simulink model "feedbackLin_Sensores_Noise"  (R2021a)
settings: Solver=ode1  StartTime=00  StopTime=100  FixedStep=0.005  RelTol=1e-3
values from neighbouring files (symbols this model uses):
  g = 9.31    [Metrics_Info.m]    (also in initEnv.m)
undefined symbols (not defined in the file or in its folder): Controller, DiscIntNeverNeededParam, Discrete, Earth, Estimator, gcbh, init, Rec, rho, SDTV, sensorCalibrationData, Sensors, States, Time, Ts, var_acc_angle_N, var_bias_gyr_N, var_gyro_p_N, Vehicle, vrmfunc, VTs, WGS84
libraries: simulink x26, ctrlSharedLib x4, sharedtransform x3, shared6dof x1, aerolibasang x1, dynamicsLibrary x1, aerolibtransform2 x1, aerolibnav x1, visionconversions x1, visiongeotforms x1
(part 2 of 3)

== system feedbackLin_Sensores_Noise/Subsystem2/Subsystem/State Estimator/SensorPreprocessing/sensordata_group ==
  HAL_acc_SI : Inport  OutDataTypeStr=Bus: HAL_acc_SI_t
  HAL_gyro_SI : Inport  Port=2  OutDataTypeStr=Bus: HAL_gyro_SI_t
  HAL_ultrasound_SI : Inport  Port=3  OutDataTypeStr=Bus: HAL_ultrasound_SI_t
  HAL_pressure_SI : Inport  Port=4  OutDataTypeStr=Bus: HAL_pressure_SI_t
  HAL_vbat_SI : Inport  Port=5  OutDataTypeStr=Bus: HAL_vbat_SI_t
  Bus Selector1 : BusSelector  OutputSignals=vbat_V,vbat_percentage
  Bus Selector3 : BusSelector  OutputSignals=x,y,z
  Bus Selector4 : BusSelector  OutputSignals=x,y,z,temperature
  Bus Selector5 : BusSelector  OutputSignals=altitude
  Bus Selector6 : BusSelector  OutputSignals=pressure
  Out Bus Element : Outport  VectorParamsAs1DForOutWhenUnconnected=off  PortName=sensordata_datin  Element=ddx
  Out Bus Element1 : Outport  VectorParamsAs1DForOutWhenUnconnected=off  PortName=sensordata_datin  Element=ddy
  Out Bus Element2 : Outport  VectorParamsAs1DForOutWhenUnconnected=off  PortName=sensordata_datin  Element=ddz
  Out Bus Element3 : Outport  VectorParamsAs1DForOutWhenUnconnected=off  PortName=sensordata_datin  Element=p
  Out Bus Element4 : Outport  VectorParamsAs1DForOutWhenUnconnected=off  PortName=sensordata_datin  Element=q
  Out Bus Element5 : Outport  VectorParamsAs1DForOutWhenUnconnected=off  PortName=sensordata_datin  Element=r
  Out Bus Element6 : Outport  VectorParamsAs1DForOutWhenUnconnected=off  PortName=sensordata_datin  Element=altitude_sonar
  Out Bus Element7 : Outport  VectorParamsAs1DForOutWhenUnconnected=off  PortName=sensordata_datin  Element=prs
  Out Bus Element8 : Outport  VectorParamsAs1DForOutWhenUnconnected=off  PortName=sensordata_datin  Element=vbat_V
  Out Bus Element9 : Outport  VectorParamsAs1DForOutWhenUnconnected=off  PortName=sensordata_datin  Element=vbat_percentage
  Out1 : Outport  Port=2
  wires:
  HAL_gyro_SI/1 -> Bus Selector4/1
  HAL_acc_SI/1 -> Bus Selector3/1
  HAL_pressure_SI/1 -> Bus Selector6/1
  HAL_ultrasound_SI/1 -> Bus Selector5/1
  Bus Selector4/1 -> Out Bus Element3/1  "<x>"
  Bus Selector3/3 -> Out Bus Element2/1  "<z>"
  Bus Selector4/3 -> Out Bus Element5/1  "<z>"
  Bus Selector5/1 -> Out Bus Element6/1  "<altitude>"
  Bus Selector6/1 -> Out Bus Element7/1  "<pressure>"
  Bus Selector4/2 -> Out Bus Element4/1  "<y>"
  Bus Selector3/1 -> Out Bus Element/1  "<x>"
  Bus Selector3/2 -> Out Bus Element1/1  "<y>"
  Bus Selector1/1 -> Out Bus Element8/1  "<vbat_V>"
  HAL_vbat_SI/1 -> Bus Selector1/1
  Bus Selector1/2 -> Out Bus Element9/1  "<vbat_percentage>"
  Bus Selector4/4 -> Out1/1  "<temperature>"

== system feedbackLin_Sensores_Noise/Subsystem2/Subsystem/State Estimator/XY Position Estimator/EstimatorVelocity ==
  opticalFlow_datin : Inport
  Z_estimin : Inport  Port=2  SampleTime=Ts
  sensorIMU_datin : Inport  Port=3
  orient_estimin : Inport  Port=4
  angular velocity : Inport  Port=5
  AccelerationHandling : Subsystem
  Angular velocity compensation for optical flow : Subsystem
  DataHandling : Subsystem
  Delay : Delay  DelayLength=1  InitialCondition=0
  KalmanFilter_dxdy : ctrlSharedLib/Kalman Filter  TimeDomain=Discrete-Time  UseCurrentEstimator=on  ModelSource=Individual A, B, C, D matrices  ModelSourceVariable=ss(0.95,1,1,0,1)  A=Estimator.pos.kfVelo.A  B=Estimator.pos.kfVelo.B  C=Estimator.pos.kfVelo.C  D=Estimator.pos.kfVelo.D  NumberOfStates=1  NumberOfInputs=1  NumberOfOutputs=1  InitialEstimateSource=Dialog  X0=0  P0=10  UseK=off  UseGH=off  NumberOfProcessNoiseInputs=1  G=Estimator.pos.kfVelo.G  TimeInvariantG=on  H=Estimator.pos.kfVelo.H  TimeInvariantH=on  Q=Estimator.pos.kfVelo.Q  TimeInvariantQ=on  R=Estimator.pos.kfVelo.R  TimeInvariantR=on  N=Estimator.pos.kfVelo.N  TimeInvariantN=on  AddInputPort=on  AddEnablePort=on  OutputEstimatedY=off  OutputP=off  Ts=-1
  Selector1 : Selector  InputPortWidth=4  IndexOptions=Index vector (dialog)  Indices=[1 2]  OutputSizes=1
  XY velocity w/o angular velocity compensation : Subsystem
  Z_estimin1 : InportShadow  Port=2  SampleTime=Ts
  angular velocity compensation : Sum
  dxy_estimout : Outport  VectorParamsAs1DForOutWhenUnconnected=off
  wires:
  Z_estimin/1 -> DataHandling/1(Z_estimin), AccelerationHandling/4(Z_estimin)
  KalmanFilter_dxdy/1 -> Selector1/1
  sensorIMU_datin/1 -> AccelerationHandling/2(sensorIMU_datin), DataHandling/3(sensorIMU_datin)
  orient_estimin/1 -> AccelerationHandling/3(orient_estimin), DataHandling/2(orient_estimin)
  Z_estimin1/1 -> XY velocity w/o angular velocity compensation/2(z_estimate), Angular velocity compensation for optical flow/1(z_estimate)
  AccelerationHandling/1(acceleration_world) -> KalmanFilter_dxdy/1
  angular velocity compensation/1 -> KalmanFilter_dxdy/2
  Delay/1 -> DataHandling/5(dxyOF_datin)
  Selector1/1 -> dxy_estimout/1, Delay/1
  angular velocity/1 -> Angular velocity compensation for optical flow/2(Angular velocity w/o bias)
  Angular velocity compensation for optical flow/1(angular velocity correction) -> angular velocity compensation/2
  XY velocity w/o angular velocity compensation/1(optical_flow_dx_dy) -> DataHandling/4(dxy_estimin), AccelerationHandling/1(dxy_estimin), angular velocity compensation/1
  opticalFlow_datin/1 -> XY velocity w/o angular velocity compensation/1(optical_flow)
  DataHandling/1(enable_flag) -> KalmanFilter_dxdy/3

== system feedbackLin_Sensores_Noise/Subsystem2/Subsystem/State Estimator/XY Position Estimator/EstimatorXYPosition ==
  note: Switching from orientationControl to Position
      | control reset the current world position estimate
      | (happens when using no markers)
  dxy_estimin : Inport
  orient_estimin : Inport  Port=2  SampleTime=Ts
  controlModePosVSOrient_flagin : Inport  Port=3
  dz_estimin : Inport  Port=4
  Math Function : Math  Operator=transpose  SignedPower=on  SaturateOnIntegerOverflow=on
  Mux2 : Mux  Inputs=2
  Product : Product  Multiplication=Matrix(*)
  Rotation Angles to Direction Cosine Matrix : sharedtransform/Rotation Angles to Direction Cosine Matrix  rotationOrder=ZYX  aMode=aMode
      settings: SourceProductBaseCode=AE,PW,DR,MT,UV,VE
  Scope : Scope
  SelectdXY : Selector  InputPortWidth=3  IndexOptions=Index vector (dialog)  Indices=[1 2]  OutputSizes=1
  SimplyIntegrateVelocity : DiscreteIntegrator  ExternalReset=rising  SampleTime=Ts  ICPrevOutput=DiscIntNeverNeededParam  ICPrevScaledInput=DiscIntNeverNeededParam
  XY_estimout : Outport  VectorParamsAs1DForOutWhenUnconnected=off
  wires:
  controlModePosVSOrient_flagin/1 -> SimplyIntegrateVelocity/2
  Product/1 -> SelectdXY/1
  Mux2/1 -> Product/2
  dz_estimin/1 -> Mux2/2
  SimplyIntegrateVelocity/1 -> XY_estimout/1
  dxy_estimin/1 -> Mux2/1
  orient_estimin/1 -> Rotation Angles to Direction Cosine Matrix/1
  Rotation Angles to Direction Cosine Matrix/1 -> Math Function/1
  SelectdXY/1 -> Scope/1, SimplyIntegrateVelocity/1
  Math Function/1 -> Product/1

== system feedbackLin_Sensores_Noise/Subsystem2/Subsystem/Sensors Model/Sensors (Dynamics)/Sensor System/Camera ==
  note: Optical flow is measured by using a camera and is calculated based on how the image actually moves. It is thus dependant on body angular velocity and body's linear velocity.
  note: This is a crude simulation of "optical flow" (vx,vy,vz) as
      | fed into the c-function rsedu_optical_flow() on the Rolling Spider
      | by internal, inaccessible code of Parrot's firmware.
      | This is assumed to be far from what "optical flow (vx,vy,vz)" actually is!
  states : Inport  OutDataTypeStr=Bus: StatesBus
  Add1 : Sum
  Bus Selector1 : BusSelector  OutputSignals=V_body
  Bus Selector3 : BusSelector  OutputSignals=X_ned
  Bus Selector4 : BusSelector  OutputSignals=Omega_body
  Data Type Conversion : DataTypeConversion  OutDataTypeStr=single
  Demux4 : Demux  Outputs=2
  Divide : Product  Inputs=*/
  Gain1 : Gain  Gain=0.8*[-1,1]
  Gain2 : Gain  Gain=-1
  Mux7 : Mux  Inputs=2
  Mux8 : Mux  Inputs=2
  Product : Product
  Product1 : Product
  Reshape : Reshape
  Select dx,dy : Selector  InputPortWidth=3  IndexOptions=Index vector (dialog)  Indices=[1 2]  OutputSizes=1
  Select dx,dy1 : Selector  InputPortWidth=3  IndexOptions=Index vector (dialog)  Indices=[1 2]  OutputSizes=1
  Select dz : Selector  InputPortWidth=3  IndexOptions=Index vector (dialog)  Indices=3  OutputSizes=1
  Select dz1 : Selector  InputPortWidth=3  IndexOptions=Index vector (dialog)  Indices=3  OutputSizes=1
  SwitchPlanarOpticalFlow : Selector  InputPortWidth=2  IndexOptions=Index vector (dialog)  Indices=[2 1]  OutputSizes=1
  VelocityToOpticalFlow_Gain : Gain  Gain=Sensors.velocityToOpticalFlowGain
  opticalFlow_datout : Outport  VectorParamsAs1DForOutWhenUnconnected=off
  wires:
  SwitchPlanarOpticalFlow/1 -> Add1/2
  Select dz/1 -> Mux8/2
  Bus Selector3/1 -> Select dz1/1  "<X_ned>"
  Mux7/1 -> SwitchPlanarOpticalFlow/1
  Bus Selector4/1 -> Reshape/1  "<Omega_body>"
  VelocityToOpticalFlow_Gain/1 -> Data Type Conversion/1
  Select dx,dy/1 -> Add1/1
  Reshape/1 -> Select dx,dy1/1
  Data Type Conversion/1 -> opticalFlow_datout/1
  Gain2/1 -> Divide/2, Product1/2, Product/2
  Divide/1 -> Mux8/1
  Product1/1 -> Mux7/2
  Select dx,dy1/1 -> Gain1/1
  Product/1 -> Mux7/1
  Demux4/1 -> Product/1
  Gain1/1 -> Demux4/1
  Select dz1/1 -> Gain2/1
  Bus Selector1/1 -> Select dz/1, Select dx,dy/1  "<V_body>"
  Demux4/2 -> Product1/1
  Mux8/1 -> VelocityToOpticalFlow_Gain/1
  states/1 -> Bus Selector1/1, Bus Selector4/1, Bus Selector3/1
  Add1/1 -> Divide/1

== system feedbackLin_Sensores_Noise/Subsystem2/Subsystem/Sensors Model/Sensors (Dynamics)/Sensor System/IMU_Pressure ==
  note: IMU block simulates the 6DOF sensor MPU6050 that we have on board. Please note that this model cannot simulate the gyro's bias change over time!
  States : Inport
  Environment : Inport  Port=2
  Assumes takeoff was level1 : Bias  Bias=Sensors.altToPrsBias
  Bus Selector : BusSelector  OutputSignals=Accel_body,Omega_body,dOmega_body,DCM_be,X_ned
  Bus Selector1 : BusSelector  OutputSignals=Gravity_ned
  CG location : Constant  Value=Sensors.IMU.cg
  Data Type Conversion{,1..4} (5 alike) : DataTypeConversion  OutDataTypeStr=single
  Demux : Demux  Outputs=3
  Demux2 : Demux  Outputs=3
  HAL_acquisition_creator : Subsystem
  Mux : Mux  Inputs=8
  Product : Product  Multiplication=Matrix(*)
  Saturation : Saturate  UpperLimit=inf  LowerLimit=Sensors.altSensorMin  OutDataTypeStr=single
  Selector2 : Selector  InputPortWidth=3  IndexOptions=Index vector (dialog)  Indices=[3]  OutputSizes=1
  Three-axis Inertial Measurement Unit : aerolibnav/Three-axis Inertial Measurement Unit  units=Metric (MKS)  imu=Sensors.IMU.location  i_Ts=Ts  dtype_a=off  w_a=.7  z_a=.2  a_sf_cc=Sensors.IMU.accScaleCross  a_bias=Sensors.IMU.accBias  a_sat=Sensors.IMU.accLimits  dtype_g=off  w_g=.7  z_g=.2  g_sf_cc=Sensors.IMU.gyroScaleCross  g_bias=Sensors.IMU.gyroBias  g_sens=Sensors.IMU.gyroGBias  g_sat=Sensors.IMU.gyroLimits  i_rand=on  i_seeds=Sensors.IMU.noiseSeeds  i_pow=Sensors.IMU.noisePower
  altToprs_gain : Gain  Gain=Sensors.altToPrsGain  ParamDataTypeStr=single  OutDataTypeStr=single
  altToprs_gain1 : Gain  Gain=-1  ParamDataTypeStr=single  OutDataTypeStr=single
  sensordata_datout : Outport  OutDataTypeStr=Bus: HAL_acquisition_t  VectorParamsAs1DForOutWhenUnconnected=off
  wires:
  altToprs_gain1/1 -> Saturation/1
  Data Type Conversion4/1 -> Mux/8
  Data Type Conversion3/1 -> Mux/7
  Data Type Conversion2/1 -> Demux2/1
  Data Type Conversion/1 -> Demux/1
  Assumes takeoff was level1/1 -> Data Type Conversion4/1
  Bus Selector/5 -> Selector2/1  "<X_ned>"
  States/1 -> Bus Selector/1
  Product/1 -> Three-axis Inertial Measurement Unit/5
  Bus Selector1/1 -> Product/2  "<Gravity_ned>"
  Bus Selector/4 -> Product/1  "<DCM_be>"
  CG location/1 -> Three-axis Inertial Measurement Unit/4
  Bus Selector/3 -> Three-axis Inertial Measurement Unit/3  "<dOmega_body>"
  Environment/1 -> Bus Selector1/1
  Bus Selector/2 -> Three-axis Inertial Measurement Unit/2  "<Omega_body>"
  Bus Selector/1 -> Three-axis Inertial Measurement Unit/1  "<Accel_body>"
  HAL_acquisition_creator/1(HAL_acquisition_t) -> sensordata_datout/1
  Data Type Conversion1/1 -> HAL_acquisition_creator/1(sensors)
  Three-axis Inertial Measurement Unit/2 -> Data Type Conversion2/1
  Three-axis Inertial Measurement Unit/1 -> Data Type Conversion/1
  Mux/1 -> Data Type Conversion1/1
  altToprs_gain/1 -> Assumes takeoff was level1/1  "prs"
  Saturation/1 -> Data Type Conversion3/1  "altitude_sonar"
  Selector2/1 -> altToprs_gain/1, altToprs_gain1/1
  Demux/3 -> Mux/3  "ddz"
  Demux2/3 -> Mux/6  "r"
  Demux/2 -> Mux/2  "ddy"
  Demux/1 -> Mux/1  "ddx"
  Demux2/1 -> Mux/4  "p"
  Demux2/2 -> Mux/5  "q"

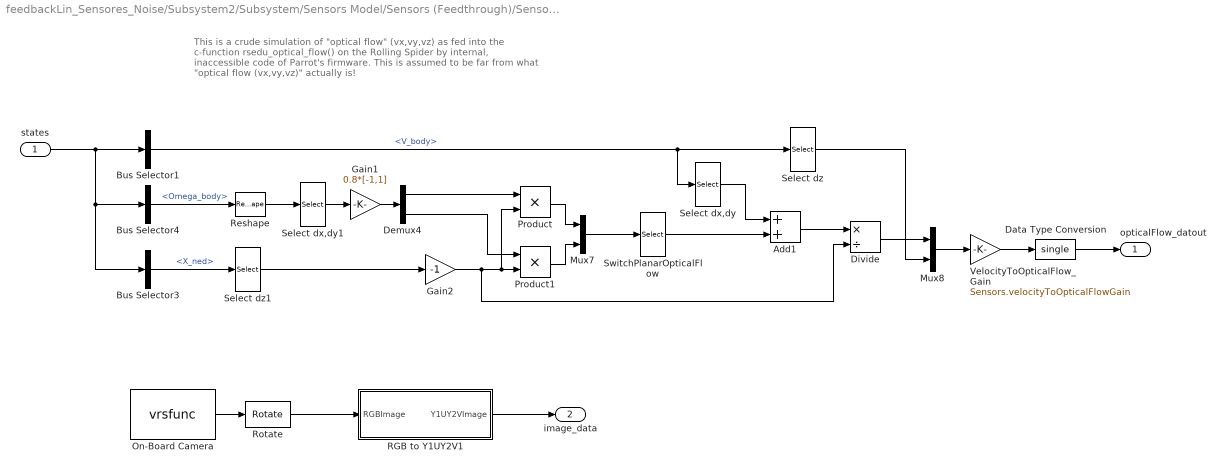
== system feedbackLin_Sensores_Noise/Subsystem2/Subsystem/Sensors Model/Sensors (Feedthrough)/Sensor System/Camera ==
  note: This is a crude simulation of "optical flow" (vx,vy,vz) as
      | fed into the c-function rsedu_optical_flow() on the Rolling Spider
      | by internal, inaccessible code of Parrot's firmware.
      | This is assumed to be far from what "optical flow (vx,vy,vz)" actually is!
  states : Inport  OutDataTypeStr=Bus: StatesBus
  Add1 : Sum
  Bus Selector1 : BusSelector  OutputSignals=V_body
  Bus Selector3 : BusSelector  OutputSignals=X_ned
  Bus Selector4 : BusSelector  OutputSignals=Omega_body
  Data Type Conversion : DataTypeConversion  OutDataTypeStr=single
  Demux4 : Demux  Outputs=2
  Divide : Product  Inputs=*/
  Gain1 : Gain  Gain=0.8*[-1,1]
  Gain2 : Gain  Gain=-1
  Mux7 : Mux  Inputs=2
  Mux8 : Mux  Inputs=2
  On-Board Camera : S-Function  InstantiateOnLoad=on  LoadFcn=vrmfunc('FnLoad', gcbh);  InitFcn=""  StartFcn=vrmfunc('FnSimStatus', gcbh, 'running')  StopFcn=vrmfunc('FnStop', gcbh)  FunctionName=vrsfunc  Parameters=SampleTime, VideoDimensions, false  SFunctionDeploymentMode=off  EnableBusSupport=off  mask(Virtual Reality Sink){SampleTime=VTs, ViewEnable=on, RemoteChange=off, RemoteView=off, FieldsWritten=, WorldFileName=asbQuadcopterWorld.wrl, WorldDescription=, AutoView=off, VideoDimensions=[160 120], AllowVariableSize=off, FigureProperties=}
      mask prompts: SampleTime "Sample Time"; ViewEnable "View"; RemoteChange "Remote Change"; RemoteView "Remote View"; FieldsWritten "Fields Written"; WorldFileName "World File Name"; WorldDescription "World Description"; VideoDimensions "Video Dimensions"; AllowVariableSize "Allow Variable Size"; FigureProperties "Figure Properties"
      mask help: Controls the selected fields of a virtual world according to given inputs.
      mask init:
      | set_param(gcbh, 'MaskDisplay', vrmfunc('FnIcon'));
      settings: CopyFcn=vrmfunc('FnCopy', gcbh);  DeleteFcn=vrmfunc('FnDelete', gcbh);  PreSaveFcn=vrmfunc('FnPreSave', gcbh);  PauseFcn=vrmfunc('FnSimStatus', gcbh, 'paused');  ContinueFcn=vrmfunc('FnSimStatus', gcbh, 'running');  DestroyFcn=vrmfunc('FnDestroy', gcbh);  OpenFcn=vrmfunc('FnOpen', gcbh);  CloseFcn=vrmfunc('FnClose', gcbh);
      mask Help: helpview(vrmfunc('FnHelpTopic'), 'vr_vrtovideo');
      mask Display: image(imread('vrblockicon.png'));
  Product : Product
  Product1 : Product
  RGB to Y1UY2V1 : Subsystem
  Reshape : Reshape
  Rotate : visiongeotforms/Rotate  outSizeR=Expanded to fit rotated input image  src_angle=Specify via dialog  unit_angle=Degrees  angle=pi/2  maxAngle=pi  dispImage=Top-left corner  method=Table lookup  fillVal=0  interpMethod=Bilinear  roundingMode=Nearest  overflowMode=on  prodOutputMode=Binary point scaling  prodOutputWordLength=32  prodOutputFracLength=10
  Select dx,dy : Selector  InputPortWidth=3  IndexOptions=Index vector (dialog)  Indices=[1 2]  OutputSizes=1
  Select dx,dy1 : Selector  InputPortWidth=3  IndexOptions=Index vector (dialog)  Indices=[1 2]  OutputSizes=1
  Select dz : Selector  InputPortWidth=3  IndexOptions=Index vector (dialog)  Indices=3  OutputSizes=1
  Select dz1 : Selector  InputPortWidth=3  IndexOptions=Index vector (dialog)  Indices=3  OutputSizes=1
  SwitchPlanarOpticalFlow : Selector  InputPortWidth=2  IndexOptions=Index vector (dialog)  Indices=[2 1]  OutputSizes=1
  VelocityToOpticalFlow_Gain : Gain  Gain=Sensors.velocityToOpticalFlowGain
  opticalFlow_datout : Outport  VectorParamsAs1DForOutWhenUnconnected=off
  image_data : Outport  Port=2  VectorParamsAs1DForOutWhenUnconnected=off
  wires:
  states/1 -> Bus Selector1/1, Bus Selector4/1, Bus Selector3/1
  Demux4/2 -> Product1/1
  Demux4/1 -> Product/1
  Bus Selector1/1 -> Select dz/1, Select dx,dy/1  "<V_body>"
  Rotate/1 -> RGB to Y1UY2V1/1(RGBImage)
  Gain1/1 -> Demux4/1
  Add1/1 -> Divide/1
  Product/1 -> Mux7/1
  Select dz1/1 -> Gain2/1
  On-Board Camera/1 -> Rotate/1
  Select dx,dy1/1 -> Gain1/1
  Gain2/1 -> Divide/2, Product1/2, Product/2
  Reshape/1 -> Select dx,dy1/1
  Divide/1 -> Mux8/1
  Data Type Conversion/1 -> opticalFlow_datout/1
  RGB to Y1UY2V1/1(Y1UY2VImage) -> image_data/1
  VelocityToOpticalFlow_Gain/1 -> Data Type Conversion/1
  Product1/1 -> Mux7/2
  Mux7/1 -> SwitchPlanarOpticalFlow/1
  Mux8/1 -> VelocityToOpticalFlow_Gain/1
  Select dx,dy/1 -> Add1/1
  Bus Selector4/1 -> Reshape/1  "<Omega_body>"
  Select dz/1 -> Mux8/2
  Bus Selector3/1 -> Select dz1/1  "<X_ned>"
  SwitchPlanarOpticalFlow/1 -> Add1/2

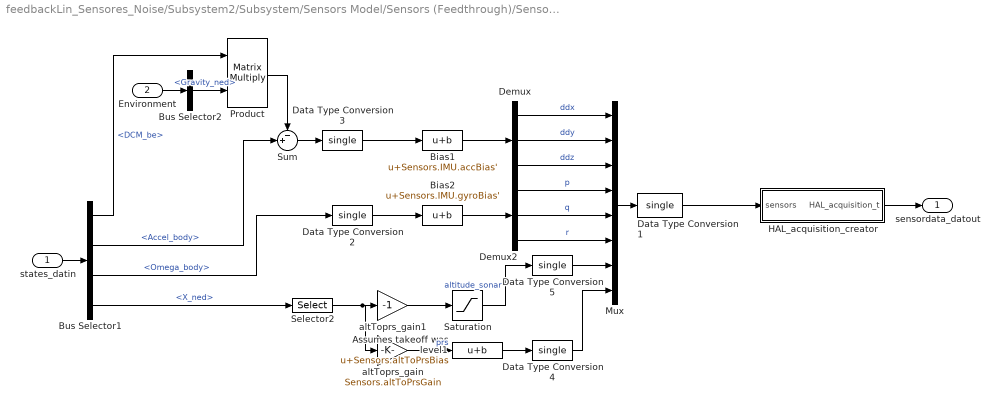
== system feedbackLin_Sensores_Noise/Subsystem2/Subsystem/Sensors Model/Sensors (Feedthrough)/Sensor System/IMU_Pressure ==
  states_datin : Inport  OutDataTypeStr=Bus: StatesBus
  Environment : Inport  Port=2
  Assumes takeoff was level1 : Bias  Bias=Sensors.altToPrsBias
  Bias1 : Bias  Bias=Sensors.IMU.accBias'
  Bias2 : Bias  Bias=Sensors.IMU.gyroBias'
  Bus Selector1 : BusSelector  OutputSignals=DCM_be,Accel_body,Omega_body,X_ned
  Bus Selector2 : BusSelector  OutputSignals=Gravity_ned
  Data Type Conversion{1..5} (5 alike) : DataTypeConversion  OutDataTypeStr=single
  Demux : Demux  Outputs=3
  Demux2 : Demux  Outputs=3
  HAL_acquisition_creator : Subsystem
  Mux : Mux  Inputs=8
  Product : Product  Multiplication=Matrix(*)
  Saturation : Saturate  UpperLimit=inf  LowerLimit=Sensors.altSensorMin  OutDataTypeStr=single
  Selector2 : Selector  InputPortWidth=3  IndexOptions=Index vector (dialog)  Indices=[3]  OutputSizes=1
  Sum : Sum  Inputs=-+|
  altToprs_gain : Gain  Gain=Sensors.altToPrsGain  ParamDataTypeStr=single  OutDataTypeStr=single
  altToprs_gain1 : Gain  Gain=-1  ParamDataTypeStr=single  OutDataTypeStr=single
  sensordata_datout : Outport  OutDataTypeStr=Bus: HAL_acquisition_t  VectorParamsAs1DForOutWhenUnconnected=off
  wires:
  Bias2/1 -> Demux2/1
  Bias1/1 -> Demux/1
  Product/1 -> Sum/1
  Bus Selector1/2 -> Sum/2  "<Accel_body>"
  Sum/1 -> Data Type Conversion3/1
  Bus Selector1/1 -> Product/1  "<DCM_be>"
  Bus Selector2/1 -> Product/2  "<Gravity_ned>"
  altToprs_gain1/1 -> Saturation/1
  Data Type Conversion5/1 -> Mux/7
  Data Type Conversion4/1 -> Mux/8
  Data Type Conversion2/1 -> Bias2/1
  Data Type Conversion3/1 -> Bias1/1
  Assumes takeoff was level1/1 -> Data Type Conversion4/1
  Bus Selector1/4 -> Selector2/1  "<X_ned>"
  states_datin/1 -> Bus Selector1/1
  Environment/1 -> Bus Selector2/1
  Bus Selector1/3 -> Data Type Conversion2/1  "<Omega_body>"
  HAL_acquisition_creator/1(HAL_acquisition_t) -> sensordata_datout/1
  Data Type Conversion1/1 -> HAL_acquisition_creator/1(sensors)
  Mux/1 -> Data Type Conversion1/1
  altToprs_gain/1 -> Assumes takeoff was level1/1  "prs"
  Saturation/1 -> Data Type Conversion5/1  "altitude_sonar"
  Selector2/1 -> altToprs_gain1/1, altToprs_gain/1
  Demux/3 -> Mux/3  "ddz"
  Demux2/3 -> Mux/6  "r"
  Demux/2 -> Mux/2  "ddy"
  Demux/1 -> Mux/1  "ddx"
  Demux2/1 -> Mux/4  "p"
  Demux2/2 -> Mux/5  "q"

== system feedbackLin_Sensores_Noise/Subsystem2/Subsystem/State Estimator/SensorPreprocessing/Temperature Compensation/Triggered Subsystem ==
  In1 : Inport
  Trigger : TriggerPort  TriggerType=either  VariantControl=Variant
  Out1 : Outport
  wires:
  In1/1 -> Out1/1

== system feedbackLin_Sensores_Noise/Subsystem2/Subsystem/State Estimator/XY Position Estimator/EstimatorVelocity/AccelerationHandling ==
  dxy_estimin : Inport
  sensorIMU_datin : Inport  Port=2
  orient_estimin : Inport  Port=3
  Z_estimin : Inport  Port=4
  Add : Sum  Inputs=-+
  Bus Selector1 : BusSelector  OutputSignals=ddx,ddy,ddz
  Deactivate Acceleration If OF is not used due to low altitude : simulink/Logic and Bit Operations/Compare To Constant  relop=<=  const=Estimator.pos.opticalFlowZMax  OutDataTypeStr=boolean
  Logical Operator : Logic  Operator=OR  AllPortsSameDT=off  OutDataTypeStr=boolean
  Mux6 : Mux  Inputs=3
  Product : Product  Inputs=3
  Product1 : Product  Multiplication=Matrix(*)
  Rotation Angles to Direction Cosine Matrix : sharedtransform/Rotation Angles to Direction Cosine Matrix  rotationOrder=ZYX  aMode=aMode
      settings: SourceProductBaseCode=AE,PW,DR,MT,UV,VE
  SelectPlanarddxy : Selector  InputPortWidth=3  IndexOptions=Index vector (dialog)  Indices=[1 2]  OutputSizes=1
  Selector : Selector  InputPortWidth=2  IndexOptions=Index vector (dialog)  Indices=1  OutputSizes=1
  Selector1 : Selector  InputPortWidth=2  IndexOptions=Index vector (dialog)  Indices=2  OutputSizes=1
  do not use acc if optical flow never available (Note OF@60Hz but ZOH to 200!) : simulink/Logic and Bit Operations/Compare To Constant  relop=~=  const=0  OutDataTypeStr=boolean
  do not use acc if optical flow never available (Note OF@60Hz but ZOH to 200!)1 : simulink/Logic and Bit Operations/Compare To Constant  relop=~=  const=0  OutDataTypeStr=boolean
  gainaccinput1 : Gain  OutDataTypeStr=single
  gravity : Constant  Value=[0 0 -g]
  acceleration_world : Outport  OutDataTypeStr=single  VectorParamsAs1DForOutWhenUnconnected=off
  wires:
  do not use acc if optical flow never available (Note OF@60Hz but ZOH to 200!)1/1 -> Logical Operator/2
  do not use acc if optical flow never available (Note OF@60Hz but ZOH to 200!)/1 -> Logical Operator/1
  Logical Operator/1 -> Product/1
  Selector1/1 -> do not use acc if optical flow never available (Note OF@60Hz but ZOH to 200!)1/1
  Selector/1 -> do not use acc if optical flow never available (Note OF@60Hz but ZOH to 200!)/1
  dxy_estimin/1 -> Selector1/1, Selector/1
  Product/1 -> acceleration_world/1
  Deactivate Acceleration If OF is not used due to low altitude/1 -> Product/3
  Z_estimin/1 -> Deactivate Acceleration If OF is not used due to low altitude/1
  Add/1 -> SelectPlanarddxy/1
  Product1/1 -> Add/1
  gravity/1 -> Product1/2
  SelectPlanarddxy/1 -> gainaccinput1/1
  Bus Selector1/3 -> Mux6/3  "<ddz>"
  Bus Selector1/1 -> Mux6/1  "<ddx>"
  sensorIMU_datin/1 -> Bus Selector1/1
  Mux6/1 -> Add/2
  Bus Selector1/2 -> Mux6/2  "<ddy>"
  orient_estimin/1 -> Rotation Angles to Direction Cosine Matrix/1
  Rotation Angles to Direction Cosine Matrix/1 -> Product1/1
  gainaccinput1/1 -> Product/2

== system feedbackLin_Sensores_Noise/Subsystem2/Subsystem/State Estimator/XY Position Estimator/EstimatorVelocity/Angular velocity compensation for optical flow ==
  note: Optical flow readings are affected by both linear and angular velocity of the drone. We need to subtract the effect of angular velocity before using the flow data
  z_estimate : Inport
  Angular velocity w/o bias : Inport  Port=2
  Abs : Abs
  Data Type Conversion : DataTypeConversion
  Demux : Demux  Outputs=2
  Gain1 : Gain  Gain=-1
  Mux : Mux  Inputs=2
  Selector : Selector  InputPortWidth=3  IndexOptions=Index vector (dialog)  Indices=[1 2]  OutputSizes=1
  prod : Product  Inputs=**
  angular velocity correction : Outport
  wires:
  Gain1/1 -> Mux/1
  Mux/1 -> Data Type Conversion/1
  Demux/2 -> Gain1/1
  Data Type Conversion/1 -> angular velocity correction/1
  prod/1 -> Demux/1
  z_estimate/1 -> Abs/1
  Demux/1 -> Mux/2
  Selector/1 -> prod/2
  Abs/1 -> prod/1
  Angular velocity w/o bias/1 -> Selector/1

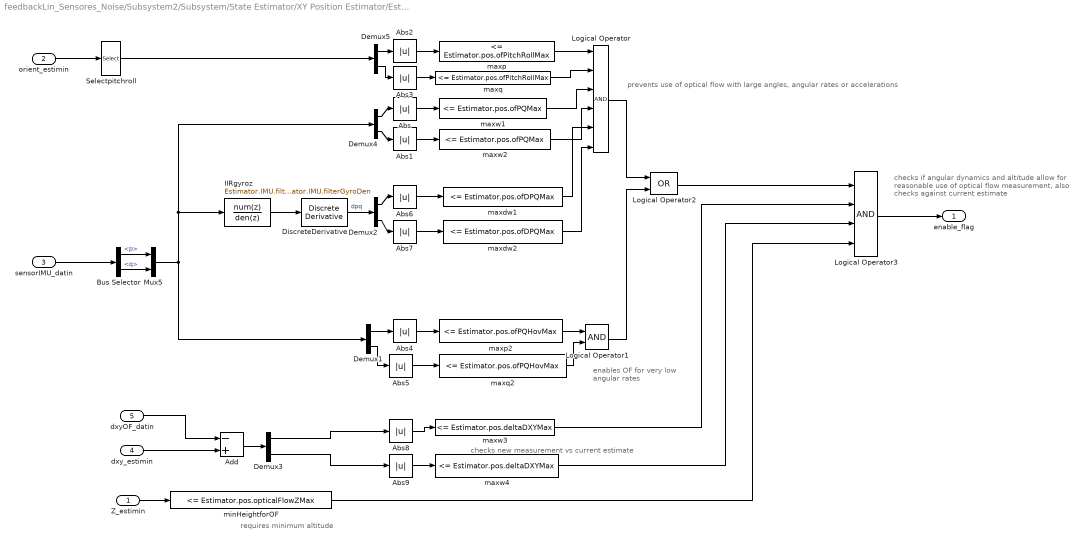
== system feedbackLin_Sensores_Noise/Subsystem2/Subsystem/State Estimator/XY Position Estimator/EstimatorVelocity/DataHandling ==
  note: prevents use of optical flow with large angles, angular rates or accelerations
  note: enables OF for very
      | low angular rates
  note: checks if angular dynamics and altitude allow for
      | reasonable use of optical flow measurement,
      | also checks against current estimate
  note: checks new measurement vs current estimate
  note: requires minimum altitude
  Z_estimin : Inport
  orient_estimin : Inport  Port=2
  sensorIMU_datin : Inport  Port=3
  dxy_estimin : Inport  Port=4
  dxyOF_datin : Inport  Port=5
  Abs{,1..9} (10 alike) : Abs
  Add : Sum  Inputs=-+
  Bus Selector : BusSelector  OutputSignals=p,q
  Demux{1..5} (5 alike) : Demux  Outputs=2
  DiscreteDerivative : simulink/Discrete/Discrete Derivative  gainval=1.0  ICPrevScaledInput=0.0  OutMin=[]  OutMax=[]  OutDataType=fixdt(1, 16)  OutScaling=2^-10  DoSatur=off
  IIRgyroz : DiscreteFilter  Numerator=Estimator.IMU.filterGyroNum  Denominator=Estimator.IMU.filterGyroDen
  Logical Operator : Logic  Inputs=6  AllPortsSameDT=off  OutDataTypeStr=boolean
  Logical Operator1 : Logic  AllPortsSameDT=off  OutDataTypeStr=boolean
  Logical Operator2 : Logic  Operator=OR  AllPortsSameDT=off  OutDataTypeStr=boolean
  Logical Operator3 : Logic  Inputs=4  AllPortsSameDT=off  OutDataTypeStr=boolean
  Mux5 : Mux  Inputs=2
  Selectpitchroll : Selector  InputPortWidth=3  IndexOptions=Index vector (dialog)  Indices=[2 3]  OutputSizes=1
  maxdw1 : simulink/Logic and Bit Operations/Compare To Constant  relop=<=  const=Estimator.pos.ofDPQMax  OutDataTypeStr=boolean
  maxdw2 : simulink/Logic and Bit Operations/Compare To Constant  relop=<=  const=Estimator.pos.ofDPQMax  OutDataTypeStr=boolean
  maxp : simulink/Logic and Bit Operations/Compare To Constant  relop=<=  const=Estimator.pos.ofPitchRollMax  OutDataTypeStr=boolean
  maxp2 : simulink/Logic and Bit Operations/Compare To Constant  relop=<=  const=Estimator.pos.ofPQHovMax  OutDataTypeStr=boolean
  maxq : simulink/Logic and Bit Operations/Compare To Constant  relop=<=  const=Estimator.pos.ofPitchRollMax  OutDataTypeStr=boolean
  maxq2 : simulink/Logic and Bit Operations/Compare To Constant  relop=<=  const=Estimator.pos.ofPQHovMax  OutDataTypeStr=boolean
  maxw1 : simulink/Logic and Bit Operations/Compare To Constant  relop=<=  const=Estimator.pos.ofPQMax  OutDataTypeStr=boolean
  maxw2 : simulink/Logic and Bit Operations/Compare To Constant  relop=<=  const=Estimator.pos.ofPQMax  OutDataTypeStr=boolean
  maxw3 : simulink/Logic and Bit Operations/Compare To Constant  relop=<=  const=Estimator.pos.deltaDXYMax  OutDataTypeStr=boolean
  maxw4 : simulink/Logic and Bit Operations/Compare To Constant  relop=<=  const=Estimator.pos.deltaDXYMax  OutDataTypeStr=boolean
  minHeightforOF : simulink/Logic and Bit Operations/Compare To Constant  relop=<=  const=Estimator.pos.opticalFlowZMax  OutDataTypeStr=boolean
  enable_flag : Outport  VectorParamsAs1DForOutWhenUnconnected=off
  wires:
  minHeightforOF/1 -> Logical Operator3/4
  IIRgyroz/1 -> DiscreteDerivative/1
  Mux5/1 -> Demux1/1, Demux4/1, IIRgyroz/1
  maxw4/1 -> Logical Operator3/3
  maxw3/1 -> Logical Operator3/2
  dxyOF_datin/1 -> Add/1
  Demux3/2 -> Abs9/1
  Demux3/1 -> Abs8/1
  dxy_estimin/1 -> Add/2
  Add/1 -> Demux3/1
  Abs9/1 -> maxw4/1
  Abs8/1 -> maxw3/1
  Logical Operator2/1 -> Logical Operator3/1
  Logical Operator3/1 -> enable_flag/1
  DiscreteDerivative/1 -> Demux2/1  "dpq"
  Demux2/2 -> Abs7/1
  Demux2/1 -> Abs6/1
  Abs7/1 -> maxdw2/1
  Abs6/1 -> maxdw1/1
  Logical Operator1/1 -> Logical Operator2/2
  Demux1/2 -> Abs5/1
  Demux1/1 -> Abs4/1
  Abs5/1 -> maxq2/1
  Abs4/1 -> maxp2/1
  Abs3/1 -> maxq/1
  Abs2/1 -> maxp/1
  Demux4/2 -> Abs1/1
  Demux4/1 -> Abs/1
  Abs1/1 -> maxw2/1
  Abs/1 -> maxw1/1
  Z_estimin/1 -> minHeightforOF/1
  Logical Operator/1 -> Logical Operator2/1
  maxw1/1 -> Logical Operator/3
  Bus Selector/1 -> Mux5/1  "<p>"
  Selectpitchroll/1 -> Demux5/1
  sensorIMU_datin/1 -> Bus Selector/1
  maxq2/1 -> Logical Operator1/2
  Bus Selector/2 -> Mux5/2  "<q>"
  maxp/1 -> Logical Operator/1
  maxw2/1 -> Logical Operator/4
  orient_estimin/1 -> Selectpitchroll/1
  maxdw1/1 -> Logical Operator/5
  maxdw2/1 -> Logical Operator/6
  maxq/1 -> Logical Operator/2
  Demux5/1 -> Abs2/1
  Demux5/2 -> Abs3/1
  maxp2/1 -> Logical Operator1/1

== system feedbackLin_Sensores_Noise/Subsystem2/Subsystem/State Estimator/XY Position Estimator/EstimatorVelocity/XY velocity w//o angular velocity compensation ==
  note: Optical flow raw readings are converted to velocity in m/s based on the estimated altitude
  optical_flow : Inport
  z_estimate : Inport  Port=2
  " " : Product  Inputs=**
  Compare To Constant : simulink/Logic and Bit Operations/Compare To Constant  relop=<  const=200*4  OutDataTypeStr=boolean
  Counter Free-Running : simulink/Sources/Counter Free-Running  NumBits=32  tsamp=-1
  Gain : Gain  Gain=-1
  Select dxy : Selector  InputPortWidth=3  IndexOptions=Index vector (dialog)  Indices=[1 2]  OutputSizes=1
  Switch : Switch  Criteria=u2 > Threshold
  opticalFlowErrorCorrect : Gain  Gain=1.15
  optical_flow_dx_dy : Outport
  wires:
  Select dxy/1 -> optical_flow_dx_dy/1  "optical_flow_dx_dy"
  " "/1 -> opticalFlowErrorCorrect/1
  opticalFlowErrorCorrect/1 -> Switch/3
  Gain/1 -> " "/2
  Switch/1 -> Select dxy/1
  Counter Free-Running/1 -> Compare To Constant/1
  Compare To Constant/1 -> Switch/2
  optical_flow/1 -> " "/1, Switch/1
  z_estimate/1 -> Gain/1

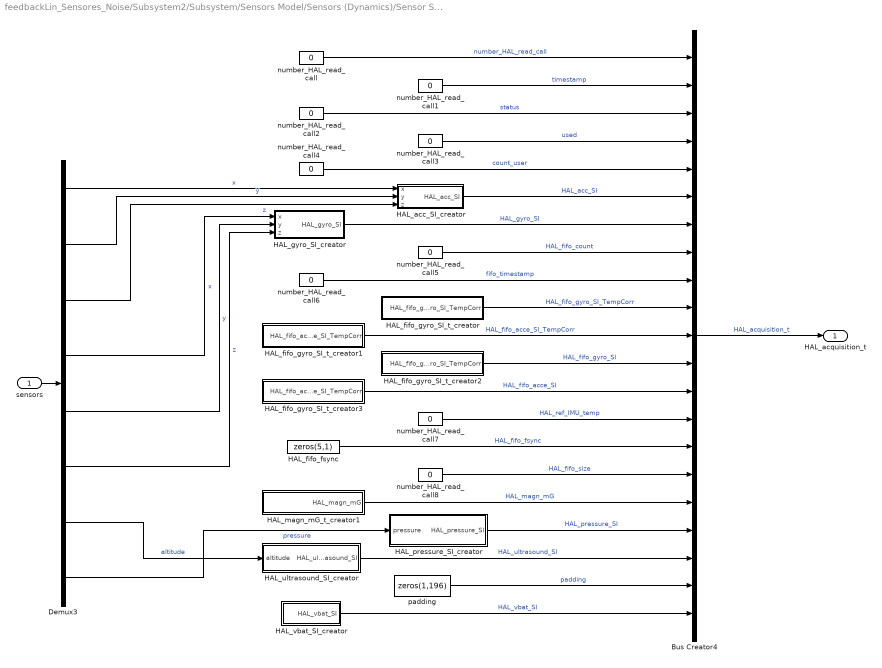
== system feedbackLin_Sensores_Noise/Subsystem2/Subsystem/Sensors Model/Sensors (Dynamics)/Sensor System/IMU_Pressure/HAL_acquisition_creator ==
  sensors : Inport
  Bus Creator4 : BusCreator  Inputs=21  OutDataTypeStr=Bus: HAL_acquisition_t  NonVirtualBus=on
      settings: InheritFromInputs=off
  Demux3 : Demux  Outputs=8
  HAL_acc_SI_creator : Subsystem
  HAL_fifo_fsync : Constant  Value=zeros(5,1)  OutDataTypeStr=uint8
  HAL_fifo_gyro_SI_t_creator : Subsystem
  HAL_fifo_gyro_SI_t_creator1 : Subsystem
  HAL_fifo_gyro_SI_t_creator2 : Subsystem
  HAL_fifo_gyro_SI_t_creator3 : Subsystem
  HAL_gyro_SI_creator : Subsystem
  HAL_magn_mG_t_creator1 : Subsystem
  HAL_pressure_SI_creator : Subsystem
  HAL_ultrasound_SI_creator : Subsystem
  HAL_vbat_SI_creator : Subsystem
  number_HAL_read_call : Constant  Value=0  OutDataTypeStr=int32
  number_HAL_read_call1 : Constant  Value=0  OutDataTypeStr=uint32
  number_HAL_read_call2 : Constant  Value=0  OutDataTypeStr=uint16
  number_HAL_read_call3 : Constant  Value=0  OutDataTypeStr=uint8
  number_HAL_read_call4 : Constant  Value=0  OutDataTypeStr=uint8
  number_HAL_read_call5 : Constant  Value=0  OutDataTypeStr=uint16
  number_HAL_read_call6 : Constant  Value=0  OutDataTypeStr=uint32
  number_HAL_read_call7 : Constant  Value=0  OutDataTypeStr=single
  number_HAL_read_call8 : Constant  Value=0  OutDataTypeStr=int32
  padding : Constant  Value=zeros(1,196)  OutDataTypeStr=uint8
  HAL_acquisition_t : Outport  OutDataTypeStr=Bus: HAL_acquisition_t  VectorParamsAs1DForOutWhenUnconnected=off
  wires:
  HAL_fifo_gyro_SI_t_creator1/1(HAL_fifo_acce_SI_TempCorr) -> Bus Creator4/11  "HAL_fifo_acce_SI_TempCorr"
  HAL_fifo_gyro_SI_t_creator2/1(HAL_fifo_gyro_SI_TempCorr) -> Bus Creator4/12  "HAL_fifo_gyro_SI"
  HAL_fifo_gyro_SI_t_creator3/1(HAL_fifo_acce_SI_TempCorr) -> Bus Creator4/13  "HAL_fifo_acce_SI"
  HAL_magn_mG_t_creator1/1(HAL_magn_mG) -> Bus Creator4/17  "HAL_magn_mG"
  HAL_fifo_fsync/1 -> Bus Creator4/15  "HAL_fifo_fsync"
  HAL_fifo_gyro_SI_t_creator/1(HAL_fifo_gyro_SI_TempCorr) -> Bus Creator4/10  "HAL_fifo_gyro_SI_TempCorr"
  number_HAL_read_call5/1 -> Bus Creator4/8  "HAL_fifo_count"
  number_HAL_read_call8/1 -> Bus Creator4/16  "HAL_fifo_size"
  number_HAL_read_call/1 -> Bus Creator4/1  "number_HAL_read_call"
  number_HAL_read_call2/1 -> Bus Creator4/3  "status"
  number_HAL_read_call3/1 -> Bus Creator4/4  "used"
  number_HAL_read_call6/1 -> Bus Creator4/9  "fifo_timestamp"
  number_HAL_read_call1/1 -> Bus Creator4/2  "timestamp"
  number_HAL_read_call4/1 -> Bus Creator4/5  "count_user"
  padding/1 -> Bus Creator4/20  "padding"
  number_HAL_read_call7/1 -> Bus Creator4/14  "HAL_ref_IMU_temp"
  HAL_vbat_SI_creator/1(HAL_vbat_SI) -> Bus Creator4/21  "HAL_vbat_SI"
  HAL_pressure_SI_creator/1(HAL_pressure_SI) -> Bus Creator4/18  "HAL_pressure_SI"
  Demux3/8 -> HAL_pressure_SI_creator/1(pressure)  "pressure"
  HAL_acc_SI_creator/1(HAL_acc_SI) -> Bus Creator4/6  "HAL_acc_SI"
  Demux3/3 -> HAL_acc_SI_creator/3(z)  "z"
  Demux3/2 -> HAL_acc_SI_creator/2(y)  "y"
  Demux3/1 -> HAL_acc_SI_creator/1(x)  "x"
  HAL_gyro_SI_creator/1(HAL_gyro_SI) -> Bus Creator4/7  "HAL_gyro_SI"
  Demux3/6 -> HAL_gyro_SI_creator/3(z)  "z"
  Demux3/5 -> HAL_gyro_SI_creator/2(y)  "y"
  Demux3/4 -> HAL_gyro_SI_creator/1(x)  "x"
  HAL_ultrasound_SI_creator/1(HAL_ultrasound_SI) -> Bus Creator4/19  "HAL_ultrasound_SI"
  Demux3/7 -> HAL_ultrasound_SI_creator/1(altitude)  "altitude"
  sensors/1 -> Demux3/1
  Bus Creator4/1 -> HAL_acquisition_t/1  "HAL_acquisition_t"

== system feedbackLin_Sensores_Noise/Subsystem2/Subsystem/Sensors Model/Sensors (Feedthrough)/Sensor System/Camera/RGB to Y1UY2V1 ==
  RGBImage : Inport  OutDataTypeStr=uint8  PortDimensions=[120 160 3]
  " RGBImage " : InportShadow  OutDataTypeStr=uint8  PortDimensions=[120 160 3]
  Blue : Selector  NumberOfDimensions=3  InputPortWidth=3  IndexOptions=Select all,Select all,Index vector (dialog)  Indices=1,1,3  OutputSizes=1,1,1
  Color Space Conversion : visionconversions/Color Space  Conversion  conversion=Obsolete  conversionActive=R'G'B' to Y'CbCr  wp_str=D65  rec=Rec. 601 (SDTV)  sys=1125/60/2:1  imagePorts=Separate color signals
  Constant : Constant  Value=1:2:120*160
  Constant1 : Constant  Value=2:2:120*160
  Constant2 : Constant  Value=1:2:120*160
  Constant3 : Constant  Value=1:2:120*160
  Green : Selector  NumberOfDimensions=3  InputPortWidth=3  IndexOptions=Select all,Select all,Index vector (dialog)  Indices=1,1,2  OutputSizes=1,1,1
  Matrix Concatenate : Concatenate  NumInputs=4  Mode=Multidimensional array
  "RGBImage " : InportShadow  OutDataTypeStr=uint8  PortDimensions=[120 160 3]
  Red : Selector  NumberOfDimensions=3  InputPortWidth=3  IndexOptions=Select all,Select all,Index vector (dialog)  Indices=1,1,1  OutputSizes=1,1,1
  Reshape1 : Reshape  OutputDimensionality=Customize  OutputDimensions=[1,19200]
  Reshape2 : Reshape  OutputDimensionality=Customize  OutputDimensions=[1,19200]
  Reshape3 : Reshape  OutputDimensionality=Customize  OutputDimensions=[1,19200]
  u : Selector  InputPortWidth=120*160  IndexOptions=Index vector (port)  Indices=[1 3]  OutputSizes=1
  v : Selector  InputPortWidth=120*160  IndexOptions=Index vector (port)  Indices=[1 3]  OutputSizes=1
  y1 : Selector  InputPortWidth=120*160  IndexOptions=Index vector (port)  Indices=[1 3]  OutputSizes=1
  y2 : Selector  InputPortWidth=120*160  IndexOptions=Index vector (port)  Indices=[1 3]  OutputSizes=1
  Y1UY2VImage : Outport  OutDataTypeStr=uint8  PortDimensions=[4 9600]  VectorParamsAs1DForOutWhenUnconnected=off
  wires:
  v/1 -> Matrix Concatenate/4
  y1/1 -> Matrix Concatenate/1
  RGBImage/1 -> Green/1
  Red/1 -> Color Space Conversion/1
  Green/1 -> Color Space Conversion/2
  Blue/1 -> Color Space Conversion/3
  Reshape3/1 -> y1/1, y2/1
  Reshape1/1 -> u/1
  Reshape2/1 -> v/1
  Constant/1 -> y1/2
  Constant1/1 -> y2/2
  Constant2/1 -> u/2
  Constant3/1 -> v/2
  Matrix Concatenate/1 -> Y1UY2VImage/1
  u/1 -> Matrix Concatenate/2
  y2/1 -> Matrix Concatenate/3
  " RGBImage "/1 -> Red/1
  "RGBImage "/1 -> Blue/1
  Color Space Conversion/1 -> Reshape3/1
  Color Space Conversion/2 -> Reshape1/1
  Color Space Conversion/3 -> Reshape2/1

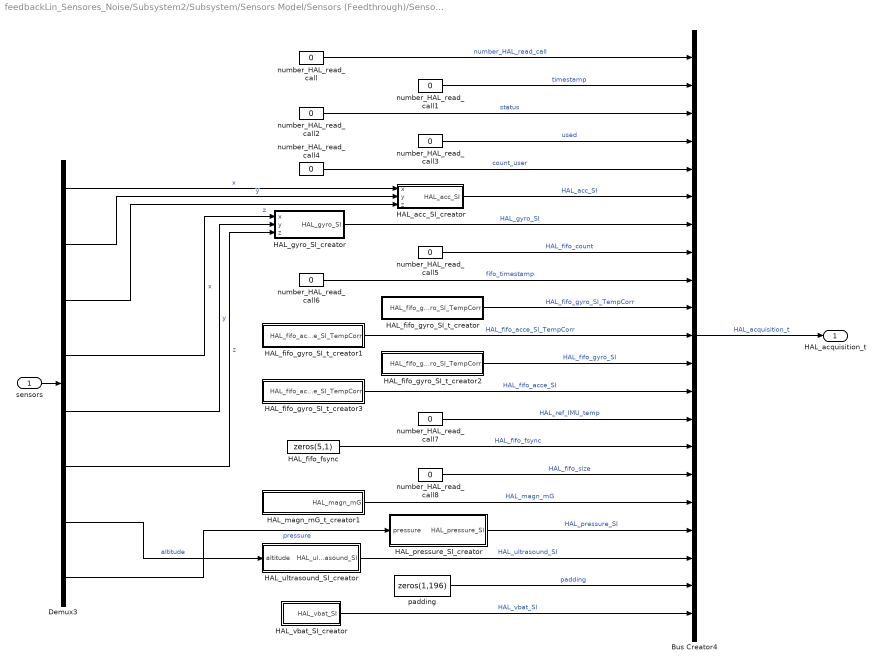
== system feedbackLin_Sensores_Noise/Subsystem2/Subsystem/Sensors Model/Sensors (Feedthrough)/Sensor System/IMU_Pressure/HAL_acquisition_creator ==
  sensors : Inport
  Bus Creator4 : BusCreator  Inputs=21  OutDataTypeStr=Bus: HAL_acquisition_t  NonVirtualBus=on
      settings: InheritFromInputs=off
  Demux3 : Demux  Outputs=8
  HAL_acc_SI_creator : Subsystem
  HAL_fifo_fsync : Constant  Value=zeros(5,1)  OutDataTypeStr=uint8
  HAL_fifo_gyro_SI_t_creator : Subsystem
  HAL_fifo_gyro_SI_t_creator1 : Subsystem
  HAL_fifo_gyro_SI_t_creator2 : Subsystem
  HAL_fifo_gyro_SI_t_creator3 : Subsystem
  HAL_gyro_SI_creator : Subsystem
  HAL_magn_mG_t_creator1 : Subsystem
  HAL_pressure_SI_creator : Subsystem
  HAL_ultrasound_SI_creator : Subsystem
  HAL_vbat_SI_creator : Subsystem
  number_HAL_read_call : Constant  Value=0  OutDataTypeStr=int32
  number_HAL_read_call1 : Constant  Value=0  OutDataTypeStr=uint32
  number_HAL_read_call2 : Constant  Value=0  OutDataTypeStr=uint16
  number_HAL_read_call3 : Constant  Value=0  OutDataTypeStr=uint8
  number_HAL_read_call4 : Constant  Value=0  OutDataTypeStr=uint8
  number_HAL_read_call5 : Constant  Value=0  OutDataTypeStr=uint16
  number_HAL_read_call6 : Constant  Value=0  OutDataTypeStr=uint32
  number_HAL_read_call7 : Constant  Value=0  OutDataTypeStr=single
  number_HAL_read_call8 : Constant  Value=0  OutDataTypeStr=int32
  padding : Constant  Value=zeros(1,196)  OutDataTypeStr=uint8
  HAL_acquisition_t : Outport  OutDataTypeStr=Bus: HAL_acquisition_t  VectorParamsAs1DForOutWhenUnconnected=off
  wires:
  HAL_fifo_gyro_SI_t_creator1/1(HAL_fifo_acce_SI_TempCorr) -> Bus Creator4/11  "HAL_fifo_acce_SI_TempCorr"
  HAL_fifo_gyro_SI_t_creator2/1(HAL_fifo_gyro_SI_TempCorr) -> Bus Creator4/12  "HAL_fifo_gyro_SI"
  HAL_fifo_gyro_SI_t_creator3/1(HAL_fifo_acce_SI_TempCorr) -> Bus Creator4/13  "HAL_fifo_acce_SI"
  HAL_magn_mG_t_creator1/1(HAL_magn_mG) -> Bus Creator4/17  "HAL_magn_mG"
  HAL_fifo_fsync/1 -> Bus Creator4/15  "HAL_fifo_fsync"
  HAL_fifo_gyro_SI_t_creator/1(HAL_fifo_gyro_SI_TempCorr) -> Bus Creator4/10  "HAL_fifo_gyro_SI_TempCorr"
  number_HAL_read_call5/1 -> Bus Creator4/8  "HAL_fifo_count"
  number_HAL_read_call8/1 -> Bus Creator4/16  "HAL_fifo_size"
  number_HAL_read_call/1 -> Bus Creator4/1  "number_HAL_read_call"
  number_HAL_read_call2/1 -> Bus Creator4/3  "status"
  number_HAL_read_call3/1 -> Bus Creator4/4  "used"
  number_HAL_read_call6/1 -> Bus Creator4/9  "fifo_timestamp"
  number_HAL_read_call1/1 -> Bus Creator4/2  "timestamp"
  number_HAL_read_call4/1 -> Bus Creator4/5  "count_user"
  padding/1 -> Bus Creator4/20  "padding"
  number_HAL_read_call7/1 -> Bus Creator4/14  "HAL_ref_IMU_temp"
  HAL_vbat_SI_creator/1(HAL_vbat_SI) -> Bus Creator4/21  "HAL_vbat_SI"
  HAL_pressure_SI_creator/1(HAL_pressure_SI) -> Bus Creator4/18  "HAL_pressure_SI"
  Demux3/8 -> HAL_pressure_SI_creator/1(pressure)  "pressure"
  HAL_acc_SI_creator/1(HAL_acc_SI) -> Bus Creator4/6  "HAL_acc_SI"
  Demux3/3 -> HAL_acc_SI_creator/3(z)  "z"
  Demux3/2 -> HAL_acc_SI_creator/2(y)  "y"
  Demux3/1 -> HAL_acc_SI_creator/1(x)  "x"
  HAL_gyro_SI_creator/1(HAL_gyro_SI) -> Bus Creator4/7  "HAL_gyro_SI"
  Demux3/6 -> HAL_gyro_SI_creator/3(z)  "z"
  Demux3/5 -> HAL_gyro_SI_creator/2(y)  "y"
  Demux3/4 -> HAL_gyro_SI_creator/1(x)  "x"
  HAL_ultrasound_SI_creator/1(HAL_ultrasound_SI) -> Bus Creator4/19  "HAL_ultrasound_SI"
  Demux3/7 -> HAL_ultrasound_SI_creator/1(altitude)  "altitude"
  sensors/1 -> Demux3/1
  Bus Creator4/1 -> HAL_acquisition_t/1  "HAL_acquisition_t"

== system feedbackLin_Sensores_Noise/Subsystem2/Subsystem/Sensors Model/Sensors (Dynamics)/Sensor System/IMU_Pressure/HAL_acquisition_creator/HAL_acc_SI_creator ==
  x : Inport
  y : Inport  Port=2
  z : Inport  Port=3
  Bus Creator : BusCreator  Inputs=4  OutDataTypeStr=Bus: HAL_acc_SI_t
  temperature : Constant  Value=0  OutDataTypeStr=single
  HAL_acc_SI : Outport  VectorParamsAs1DForOutWhenUnconnected=off
  wires:
  y/1 -> Bus Creator/2  "y"
  x/1 -> Bus Creator/1  "x"
  z/1 -> Bus Creator/3  "z"
  Bus Creator/1 -> HAL_acc_SI/1  "HAL_acc_SI"
  temperature/1 -> Bus Creator/4  "temperature"

== system feedbackLin_Sensores_Noise/Subsystem2/Subsystem/Sensors Model/Sensors (Dynamics)/Sensor System/IMU_Pressure/HAL_acquisition_creator/HAL_fifo_gyro_SI_t_creator ==
  Bus Creator : BusCreator  Inputs=3  OutDataTypeStr=Bus: HAL_fifo_gyro_SI_t  NonVirtualBus=on
      settings: InheritFromInputs=off
  Vector Concatenate : Concatenate  NumInputs=5
  z : Constant  Value=0  OutDataTypeStr=single
  z1 : Constant  Value=0  OutDataTypeStr=single
  z2 : Constant  Value=0  OutDataTypeStr=single
  HAL_fifo_gyro_SI_TempCorr : Outport  PortDimensions=5  VectorParamsAs1DForOutWhenUnconnected=off  LockScale=on
  wires:
  Vector Concatenate/1 -> HAL_fifo_gyro_SI_TempCorr/1
  Bus Creator/1 -> Vector Concatenate/3, Vector Concatenate/4, Vector Concatenate/5, Vector Concatenate/2, Vector Concatenate/1  "HAL_fifo_gyro_SI_TempCorr"
  z2/1 -> Bus Creator/1  "x"
  z/1 -> Bus Creator/3  "z"
  z1/1 -> Bus Creator/2  "y"

== system feedbackLin_Sensores_Noise/Subsystem2/Subsystem/Sensors Model/Sensors (Dynamics)/Sensor System/IMU_Pressure/HAL_acquisition_creator/HAL_fifo_gyro_SI_t_creator1 ==
  Bus Creator : BusCreator  Inputs=3  OutDataTypeStr=Bus: HAL_fifo_gyro_SI_t  NonVirtualBus=on
      settings: InheritFromInputs=off
  Vector Concatenate : Concatenate  NumInputs=5
  x : Constant  Value=0  OutDataTypeStr=single
  x1 : Constant  Value=0  OutDataTypeStr=single
  x2 : Constant  Value=0  OutDataTypeStr=single
  HAL_fifo_acce_SI_TempCorr : Outport  PortDimensions=5  VectorParamsAs1DForOutWhenUnconnected=off  LockScale=on
  wires:
  x1/1 -> Bus Creator/2  "y"
  x2/1 -> Bus Creator/3  "z"
  x/1 -> Bus Creator/1  "x"
  Bus Creator/1 -> Vector Concatenate/5, Vector Concatenate/4, Vector Concatenate/3, Vector Concatenate/2, Vector Concatenate/1  "HAL_fifo_gyro_SI_TempCorr"
  Vector Concatenate/1 -> HAL_fifo_acce_SI_TempCorr/1

== system feedbackLin_Sensores_Noise/Subsystem2/Subsystem/Sensors Model/Sensors (Dynamics)/Sensor System/IMU_Pressure/HAL_acquisition_creator/HAL_fifo_gyro_SI_t_creator2 ==
  Bus Creator : BusCreator  Inputs=3  OutDataTypeStr=Bus: HAL_fifo_gyro_SI_t  NonVirtualBus=on
      settings: InheritFromInputs=off
  Vector Concatenate : Concatenate  NumInputs=5
  z : Constant  Value=0  OutDataTypeStr=single
  z1 : Constant  Value=0  OutDataTypeStr=single
  z2 : Constant  Value=0  OutDataTypeStr=single
  HAL_fifo_gyro_SI_TempCorr : Outport  PortDimensions=5  VectorParamsAs1DForOutWhenUnconnected=off  LockScale=on
  wires:
  Vector Concatenate/1 -> HAL_fifo_gyro_SI_TempCorr/1
  Bus Creator/1 -> Vector Concatenate/3, Vector Concatenate/4, Vector Concatenate/5, Vector Concatenate/2, Vector Concatenate/1  "HAL_fifo_gyro_SI_TempCorr"
  z2/1 -> Bus Creator/1  "x"
  z/1 -> Bus Creator/3  "z"
  z1/1 -> Bus Creator/2  "y"

== system feedbackLin_Sensores_Noise/Subsystem2/Subsystem/Sensors Model/Sensors (Dynamics)/Sensor System/IMU_Pressure/HAL_acquisition_creator/HAL_fifo_gyro_SI_t_creator3 ==
  Bus Creator : BusCreator  Inputs=3  OutDataTypeStr=Bus: HAL_fifo_gyro_SI_t  NonVirtualBus=on
      settings: InheritFromInputs=off
  Vector Concatenate : Concatenate  NumInputs=5
  z : Constant  Value=0  OutDataTypeStr=single
  z1 : Constant  Value=0  OutDataTypeStr=single
  z2 : Constant  Value=0  OutDataTypeStr=single
  HAL_fifo_acce_SI_TempCorr : Outport  PortDimensions=5  VectorParamsAs1DForOutWhenUnconnected=off  LockScale=on
  wires:
  z1/1 -> Bus Creator/2  "y"
  z/1 -> Bus Creator/3  "z"
  z2/1 -> Bus Creator/1  "x"
  Bus Creator/1 -> Vector Concatenate/5, Vector Concatenate/4, Vector Concatenate/3, Vector Concatenate/2, Vector Concatenate/1  "HAL_fifo_gyro_SI_TempCorr"
  Vector Concatenate/1 -> HAL_fifo_acce_SI_TempCorr/1

== system feedbackLin_Sensores_Noise/Subsystem2/Subsystem/Sensors Model/Sensors (Dynamics)/Sensor System/IMU_Pressure/HAL_acquisition_creator/HAL_gyro_SI_creator ==
  x : Inport
  y : Inport  Port=2
  z : Inport  Port=3
  Bus Creator1 : BusCreator  Inputs=5  OutDataTypeStr=Bus: HAL_gyro_SI_t
  temperature : Constant  Value=0  OutDataTypeStr=single
  temperature_lsb : Constant  Value=0  OutDataTypeStr=int32
  HAL_gyro_SI : Outport  VectorParamsAs1DForOutWhenUnconnected=off
  wires:
  temperature/1 -> Bus Creator1/4  "temperature"
  z/1 -> Bus Creator1/3  "z"
  y/1 -> Bus Creator1/2  "y"
  x/1 -> Bus Creator1/1  "x"
  Bus Creator1/1 -> HAL_gyro_SI/1  "HAL_gyro_SI"
  temperature_lsb/1 -> Bus Creator1/5  "temperature_lsb"

== system feedbackLin_Sensores_Noise/Subsystem2/Subsystem/Sensors Model/Sensors (Dynamics)/Sensor System/IMU_Pressure/HAL_acquisition_creator/HAL_magn_mG_t_creator1 ==
  Bus Creator : BusCreator  Inputs=3  OutDataTypeStr=Bus: HAL_magn_mG_t
      settings: InheritFromInputs=off
  z : Constant  Value=0  OutDataTypeStr=single
  z1 : Constant  Value=0  OutDataTypeStr=single
  z2 : Constant  Value=0  OutDataTypeStr=single
  HAL_magn_mG : Outport  VectorParamsAs1DForOutWhenUnconnected=off
  wires:
  Bus Creator/1 -> HAL_magn_mG/1  "HAL_magn_mG"
  z1/1 -> Bus Creator/2  "y"
  z/1 -> Bus Creator/3  "z"
  z2/1 -> Bus Creator/1  "x"

== system feedbackLin_Sensores_Noise/Subsystem2/Subsystem/Sensors Model/Sensors (Dynamics)/Sensor System/IMU_Pressure/HAL_acquisition_creator/HAL_pressure_SI_creator ==
  pressure : Inport
  Bus Creator3 : BusCreator  Inputs=2  OutDataTypeStr=Bus: HAL_pressure_SI_t
  temperature : Constant  Value=0  OutDataTypeStr=double
  HAL_pressure_SI : Outport  VectorParamsAs1DForOutWhenUnconnected=off
  wires:
  pressure/1 -> Bus Creator3/2  "pressure"
  Bus Creator3/1 -> HAL_pressure_SI/1  "HAL_pressure_SI"
  temperature/1 -> Bus Creator3/1  "temperature"

== system feedbackLin_Sensores_Noise/Subsystem2/Subsystem/Sensors Model/Sensors (Dynamics)/Sensor System/IMU_Pressure/HAL_acquisition_creator/HAL_ultrasound_SI_creator ==
  altitude : Inport
  Bus Creator2 : BusCreator  Inputs=8  OutDataTypeStr=Bus: HAL_ultrasound_SI_t  NonVirtualBus=on
      settings: InheritFromInputs=off
  HAL_list_echo_t_creator : Subsystem
  HAL_list_echo_t_creator1 : Subsystem
  raw_altitude : Constant  Value=0  OutDataTypeStr=single
  raw_altitude1 : Constant  Value=0  OutDataTypeStr=uint16
  raw_altitude2 : Constant  Value=0  OutDataTypeStr=int32
  raw_altitude3 : Constant  Value=0  OutDataTypeStr=int32
  raw_altitude4 : Constant  Value=0  OutDataTypeStr=uint8
  HAL_ultrasound_SI : Outport  VectorParamsAs1DForOutWhenUnconnected=off
  wires:
  HAL_list_echo_t_creator1/1(HAL_list_echo) -> Bus Creator2/8  "HAL_list_echo_p"
  raw_altitude4/1 -> Bus Creator2/6  "new_data"
  raw_altitude/1 -> Bus Creator2/2  "raw_altitude"
  altitude/1 -> Bus Creator2/1  "altitude"
  Bus Creator2/1 -> HAL_ultrasound_SI/1  "HAL_ultrasound_SI"
  raw_altitude1/1 -> Bus Creator2/3  "nb_echo"
  raw_altitude2/1 -> Bus Creator2/4  "measure_ref"
  raw_altitude3/1 -> Bus Creator2/5  "measure_status"
  HAL_list_echo_t_creator/1(HAL_list_echo) -> Bus Creator2/7  "HAL_list_echo"

== system feedbackLin_Sensores_Noise/Subsystem2/Subsystem/Sensors Model/Sensors (Dynamics)/Sensor System/IMU_Pressure/HAL_acquisition_creator/HAL_vbat_SI_creator ==
  Bus Creator5 : BusCreator  Inputs=2  OutDataTypeStr=Bus: HAL_vbat_SI_t
  Demux4 : Demux  Outputs=2
  _DUMMY_batteryStatus : Constant  Value=Sensors.dummy.batteryStatus
  convert1 : DataTypeConversion  OutDataTypeStr=single  SaturateOnIntegerOverflow=on
  convert2 : DataTypeConversion  OutDataTypeStr=uint32  SaturateOnIntegerOverflow=on
  HAL_vbat_SI : Outport  VectorParamsAs1DForOutWhenUnconnected=off
  wires:
  Bus Creator5/1 -> HAL_vbat_SI/1  "HAL_vbat_SI"
  convert2/1 -> Bus Creator5/2  "vbat_percentage"
  convert1/1 -> Bus Creator5/1  "vbat_V"
  Demux4/2 -> convert2/1
  Demux4/1 -> convert1/1
  _DUMMY_batteryStatus/1 -> Demux4/1

== system feedbackLin_Sensores_Noise/Subsystem2/Subsystem/Sensors Model/Sensors (Feedthrough)/Sensor System/IMU_Pressure/HAL_acquisition_creator/HAL_acc_SI_creator ==
  x : Inport
  y : Inport  Port=2
  z : Inport  Port=3
  Bus Creator : BusCreator  Inputs=4  OutDataTypeStr=Bus: HAL_acc_SI_t
  temperature : Constant  Value=0  OutDataTypeStr=single
  HAL_acc_SI : Outport  VectorParamsAs1DForOutWhenUnconnected=off
  wires:
  y/1 -> Bus Creator/2  "y"
  x/1 -> Bus Creator/1  "x"
  z/1 -> Bus Creator/3  "z"
  Bus Creator/1 -> HAL_acc_SI/1  "HAL_acc_SI"
  temperature/1 -> Bus Creator/4  "temperature"

== system feedbackLin_Sensores_Noise/Subsystem2/Subsystem/Sensors Model/Sensors (Feedthrough)/Sensor System/IMU_Pressure/HAL_acquisition_creator/HAL_fifo_gyro_SI_t_creator ==
  Bus Creator : BusCreator  Inputs=3  OutDataTypeStr=Bus: HAL_fifo_gyro_SI_t  NonVirtualBus=on
      settings: InheritFromInputs=off
  Vector Concatenate : Concatenate  NumInputs=5
  z : Constant  Value=0  OutDataTypeStr=single
  z1 : Constant  Value=0  OutDataTypeStr=single
  z2 : Constant  Value=0  OutDataTypeStr=single
  HAL_fifo_gyro_SI_TempCorr : Outport  PortDimensions=5  VectorParamsAs1DForOutWhenUnconnected=off  LockScale=on
  wires:
  Vector Concatenate/1 -> HAL_fifo_gyro_SI_TempCorr/1
  Bus Creator/1 -> Vector Concatenate/3, Vector Concatenate/4, Vector Concatenate/5, Vector Concatenate/2, Vector Concatenate/1  "HAL_fifo_gyro_SI_TempCorr"
  z2/1 -> Bus Creator/1  "x"
  z/1 -> Bus Creator/3  "z"
  z1/1 -> Bus Creator/2  "y"
